simulink model "k_pod"  (R2021a)
settings: Solver=VariableStepAuto  StartTime=0.0  StopTime=3  RelTol=1e-3
settings Model: Creator=Евгений  LastModifiedBy=Евгений

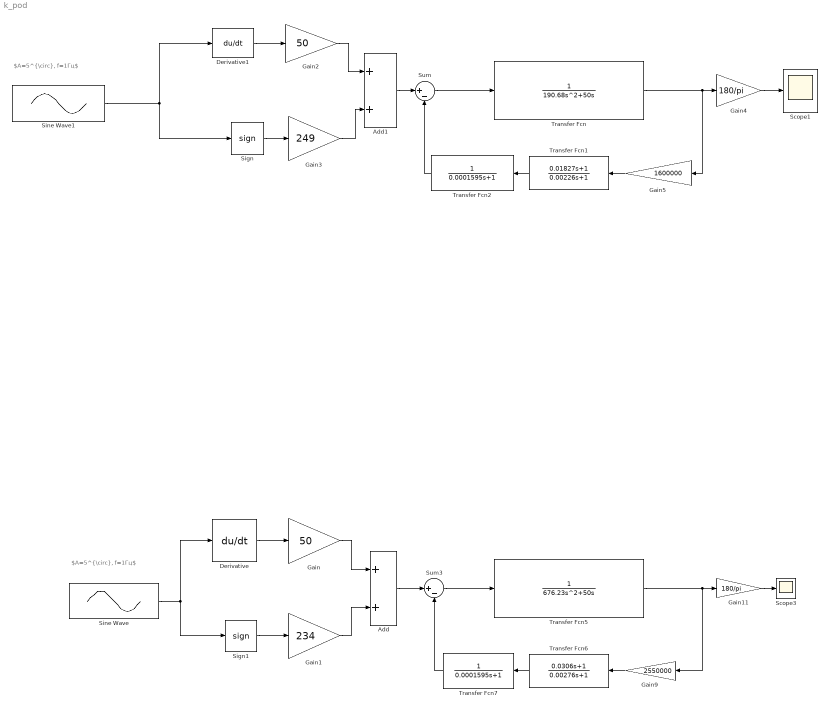
== system k_pod ==
  note: $A=5^{\circ}, f=1Гц$
  note: $A=5^{\circ}, f=1Гц$
  Add : Sum
  Add1 : Sum
  Derivative : Derivative
  Derivative1 : Derivative
  Gain : Gain  Gain=50
  Gain1 : Gain  Gain=234
  Gain11 : Gain  Gain=180/pi
  Gain2 : Gain  Gain=50
  Gain3 : Gain  Gain=249
  Gain4 : Gain  Gain=180/pi
  Gain5 : Gain  Gain=1600000
  Gain9 : Gain  Gain=2550000
  Scope1 : Scope
  Scope3 : Scope
  Sign : Signum  ZeroCross=off
  Sign1 : Signum
  Sine Wave : Sin  Amplitude=5/180*pi  Frequency=2*pi  SampleTime=0
  Sine Wave1 : Sin  Amplitude=5/180*pi  Frequency=2*pi  SampleTime=0
  Sum : Sum  Inputs=|+-
  Sum3 : Sum  Inputs=|+-
  Transfer Fcn : TransferFcn  Denominator=[190.68 50 0]
  Transfer Fcn1 : TransferFcn  Numerator="[0.01827  1]"  Denominator=[0.00226 1]
  Transfer Fcn2 : TransferFcn  Denominator=[0.0001595 1]
  Transfer Fcn5 : TransferFcn  Denominator=[676.23 50 0]
  Transfer Fcn6 : TransferFcn  Numerator="[0.0306   1]"  Denominator=[0.00276 1]
  Transfer Fcn7 : TransferFcn  Denominator="[0.0001595  1]"
  wires:
  Sine Wave/1 -> Sign1/1, Derivative/1
  Derivative/1 -> Gain/1
  Gain/1 -> Add/1
  Sign1/1 -> Gain1/1
  Gain1/1 -> Add/2
  Transfer Fcn6/1 -> Transfer Fcn7/1
  Add/1 -> Sum3/1
  Transfer Fcn7/1 -> Sum3/2
  Transfer Fcn5/1 -> Gain9/1, Gain11/1
  Sum3/1 -> Transfer Fcn5/1
  Gain9/1 -> Transfer Fcn6/1
  Gain11/1 -> Scope3/1
  Gain4/1 -> Scope1/1
  Gain3/1 -> Add1/2
  Gain2/1 -> Add1/1
  Gain5/1 -> Transfer Fcn1/1
  Transfer Fcn2/1 -> Sum/2
  Transfer Fcn1/1 -> Transfer Fcn2/1
  Sum/1 -> Transfer Fcn/1
  Transfer Fcn/1 -> Gain5/1, Gain4/1
  Add1/1 -> Sum/1
  Sign/1 -> Gain3/1
  Derivative1/1 -> Gain2/1
  Sine Wave1/1 -> Derivative1/1, Sign/1
